simulink model "gm_commrshdl_ref"  (R2023b)
settings: Solver=FixedStepDiscrete  StartTime=0.0  StopTime=2100  RelTol=1e-3
InitFcn:
  | messagelength = 32;
  | period =messagelength+672;
  | N = 255;
  | K = 223;
  | 
  | message = [212 186 161 18 242 116 150 48 39 212 136 156 150 227 169 82 179 21 171 253 146 83 7 50 192 98 72 240 25 34 224 145 98 26 193 0];
libraries: simulink x9, whdlutilities x2, whdledac x1, hdlsllib x1
settings Model: ModifiedByFormat=The MathWorks Inc.  Creator=The MathWorks, Inc.  LastModifiedBy=The MathWorks Inc.
settings SolverCC: AlgebraicLoopSolver=TrustRegion
settings DataIOCC: LimitDataPoints=on  SaveFormat=Array  SaveOutput=off  SaveTime=off  ReturnWorkspaceOutputs=off  SignalLoggingName=RS_HDL_logsout
settings OptimizationCC: BlockReduction=off  ConditionallyExecuteInputs=off  DefaultParameterBehavior=Inlined  InheritOutputTypeSmallerThanSingle=on  OptimizeBlockIOStorage=off  ExpressionDepthLimit=2147483647
settings DebuggingCC: AlgebraicLoopMsg=error  UnderspecifiedInitializationDetection=Classic  MergeDetectMultiDrivingBlocksExec=none  SolverPrmCheckMsg=warning  InheritedTsInSrcMsg=none  MultiTaskDSMMsg=warning  MultiTaskCondExecSysMsg=none  SingleTaskRateTransMsg=error  UnconnectedInputMsg=warning  UnconnectedOutputMsg=warning  UnconnectedLineMsg=warning  AllowSymbolicDim=off  StateNameClashWarn=warning  SymbolicDimsDataTypeCodeGenerationDiagnostic=none  SFUnexpectedBacktrackingDiag=warning  SFNoUnconditionalDefaultTransitionDiag=warning  SFExecutionAtInitializationDiag=none  ArithmeticOperatorsInVariantConditions=warning
settings HardwareCC: ProdBitPerPointer=32  ProdBitPerSizeT=32  ProdBitPerPtrDiffT=32  ProdLargestAtomicFloat=None  ProdIntDivRoundTo=Undefined  ProdEndianess=Unspecified  ProdWordSize=32  ProdHWDeviceType=ASIC/FPGA->ASIC/FPGA  TargetBitPerPointer=64  TargetBitPerSizeT=64  TargetBitPerPtrDiffT=64  TargetLongLongMode=on  TargetIntDivRoundTo=Zero  TargetEndianess=LittleEndian  TargetWordSize=64  TargetHWDeviceType=Generic->Custom  ProdEqTarget=off
settings ModelReferenceCC: EnableRefExpFcnMdlSchedulingChecks=on  PropagateSignalLabelsOutOfModel=off
settings SFSimCC: SimUseLocalCustomCode=off  CustomCodeUndefinedFunction=UseInterfaceOnly
settings RTWCC: Description=SystemVerilog DPI Component Generator  SystemTargetFile=systemverilog_dpi_grt.tlc  TemplateMakefile=systemverilog_dpi_grt_default_tmf  RTWVerbose=off  RTWUseLocalCustomCode=off  BuildConfiguration=Faster Runs
settings CodeAppCC: MaxIdLength=256  StateflowObjectComments=on
settings DPIGRTTargetCC: TargetFcnLib=ansi_tfl_table_tmw.mat  GenFloatMathFcnCalls=NOT IN USE  TargetLangStandard=C99 (ISO)  CodeReplacementLibrary=None  UtilityFuncGeneration=Auto  MultiwordTypeDef=System defined  MultiwordLength=2048  DynamicStringBufferSize=256  GenerateFullHeader=on  InferredTypesCompatibility=off  GenerateSampleERTMain=off  GenerateTestInterfaces=off  ModelReferenceCompliant=on  ParMdlRefBuildCompliant=on  CompOptLevelCompliant=off  ConcurrentExecutionCompliant=off  IncludeMdlTerminateFcn=on  CombineOutputUpdateFcns=off  CombineSignalStateStructs=on  GroupInternalDataByFunction=off  SuppressErrorStatus=off  IncludeFileDelimiter=Auto  ERTCustomFileBanners=off  SupportAbsoluteTime=on  LogVarNameModifier=rt_  MatFileLogging=off  CodeInterfacePackaging=Reusable function  PurelyIntegerCode=off  SupportNonFinite=on  SupportComplex=on  SupportContinuousTime=on  SupportNonInlinedSFcns=on  RemoveDisableFunc=off  RemoveResetFunc=off  SupportVariableSizeSignals=off  ParenthesesLevel=Nominal  CastingMode=Nominal  MATLABClassNameForMDSCustomization=Simulink.SoftwareTarget.TargetSpecificTriggerConfigurationBase  ModelStepFunctionPrototypeControlCompliant=off  CPPClassGenCompliant=off  AutosarCompliant=off  MDXCompliant=off  GRTInterface=off  GenerateAllocFcn=on  UseToolchainInfoCompliant=on  GenerateSharedConstants=on  CoderGroups=[]  AccessMethods=[]  LookupTableObjectStructAxisOrder=1,2,3,4,...  LUTObjectStructOrderExplicitValues=Size,Breakpoints,Table  LUTObjectStructOrderEvenSpacing=Size,Breakpoints,Table  ArrayLayout=Column-major  UnsupportedSFcnMsg=error  ERTHeaderFileRootName=$R$E  ERTSourceFileRootName=$R$E  ERTDataFileRootName=$R_data  OptimizeReductions=off  RTWCAPISignals=on  RTWCAPIParams=off  RTWCAPIStates=off  RTWCAPIRootIO=off  ExtMode=off  ExtModeTransport=0  ExtModeStaticAlloc=off  ExtModeStaticAllocSize=1000000  ExtModeTesting=off  ExtModeMexFile=ext_comm  GenerateASAP2=off  MultiInstanceErrorCode=Error  DPICustomizeSystemVerilogCode=on  DPISystemVerilogTemplate=hdlverifier_dpitb_template.vgt  DPIReportRunTimeError=off  DPIRunTimeErrorSeverity=Fatal  DPIScalarizePorts=off  DPIGenerateTestBench=off  DPITestBenchSimulator=Mentor Graphics Questasim  DPITestPointAccessFcnInterface=None  DPIFixedPointDataType=CompatibleCType  DPIPortConnection=Port list  DPICompositeDataType=Flattened  DPIComponentTemplateType=Sequential
settings ConfigComp: CovMetricSettings=dw  CovSaveCumulativeToWorkspaceVar=on  CovSaveSingleToWorkspaceVar=on  CovExternalEMLEnable=off  CovSFcnEnable=off

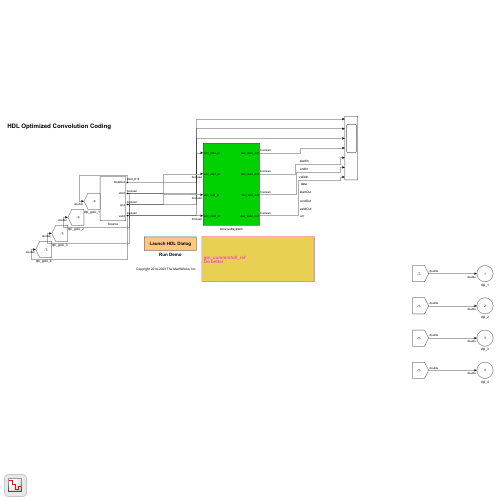
[thumbnail: Simulink's stored preview of the top-level diagram]
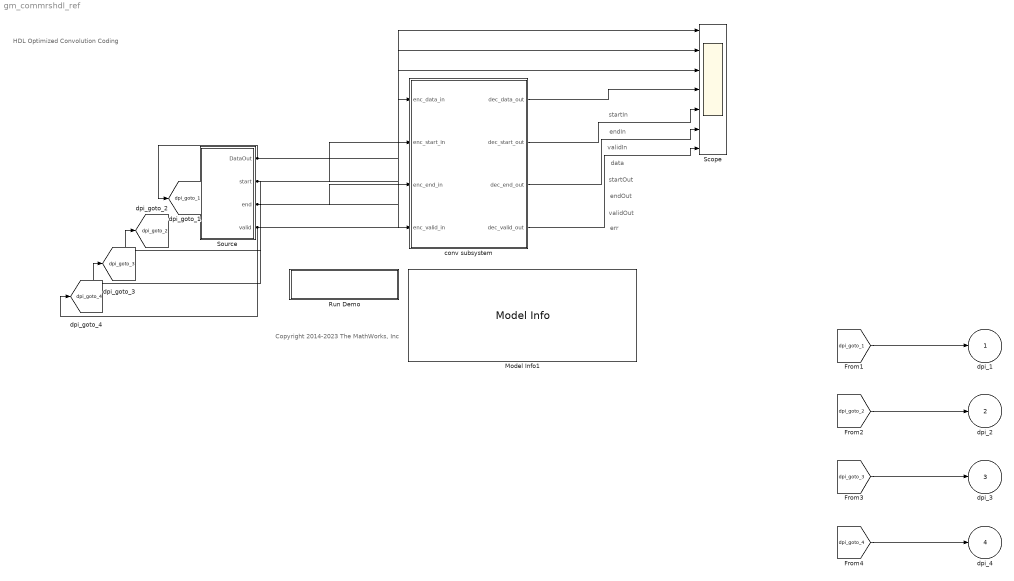
== system gm_commrshdl_ref ==
  note: err
  note: validOut
  note: endOut
  note: startOut
  note: data
  note: validIn
  note: endIn
  note: startIn
  note: Copyright 2014-2023 The MathWorks, Inc
  note: HDL Optimized Convolution Coding
  Model Info1 : simulink/Model-Wide Utilities/Model Info  Frame=on  DisplayStringWithTags=|  HorizontalTextAlignment=Left  LeftAlignmentValue=0.02
      | %<ModelName>
      | Do better
  Run Demo : Subsystem
      settings: OpenFcn=hdldialog(bdroot)
      mask Display: disp('Launch HDL Dialog')
  Scope : Scope  NumInputPorts=7
  Source : Subsystem
  conv subsystem : Subsystem
  dpi_1 : Outport
  dpi_2 : Outport  Port=2
  dpi_3 : Outport  Port=3
  dpi_4 : Outport  Port=4
  tag scope: dpi_goto_1=global, dpi_goto_2=global, dpi_goto_3=global, dpi_goto_4=global
  wires:
  Source/2(start) -> conv subsystem/2(enc_start_in), Scope/1, [dpi_goto_2]
  Source/3(end) -> conv subsystem/3(enc_end_in), Scope/2, [dpi_goto_3]
  Source/4(valid) -> conv subsystem/4(enc_valid_in), Scope/3, [dpi_goto_4]
  conv subsystem/1(dec_data_out) -> Scope/4
  conv subsystem/4(dec_valid_out) -> Scope/7
  conv subsystem/3(dec_end_out) -> Scope/6
  conv subsystem/2(dec_start_out) -> Scope/5
  Source/1(DataOut) -> conv subsystem/1(enc_data_in), [dpi_goto_1]
  [dpi_goto_1] -> dpi_1/1
  [dpi_goto_2] -> dpi_2/1
  [dpi_goto_3] -> dpi_3/1
  [dpi_goto_4] -> dpi_4/1

== system gm_commrshdl_ref/Run Demo ==

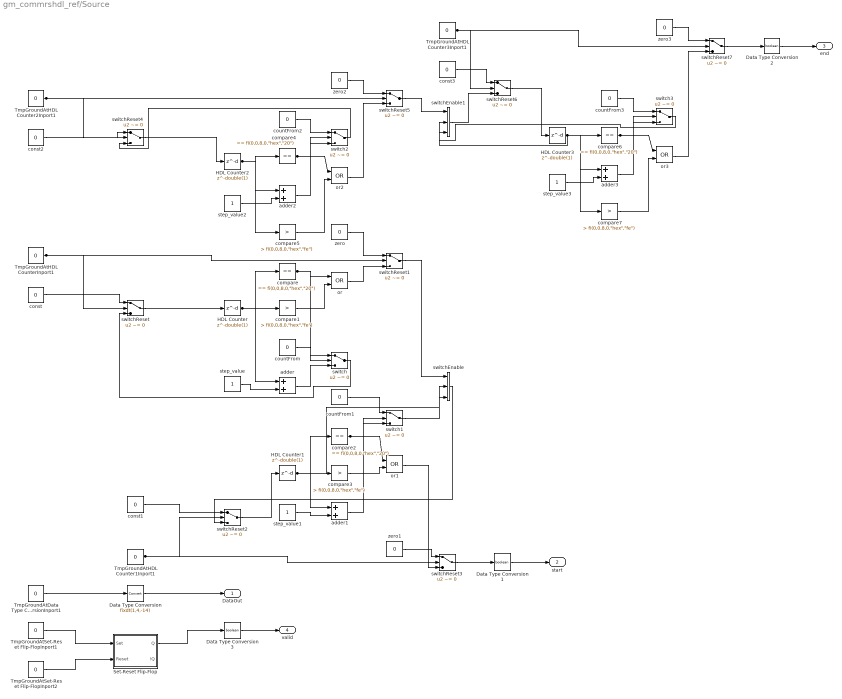
== system gm_commrshdl_ref/Source ==
  Data Type Conversion : DataTypeConversion  OutDataTypeStr=fixdt(1,4,-14)
  Data Type Conversion1 : DataTypeConversion  OutDataTypeStr=boolean
  Data Type Conversion2 : DataTypeConversion  OutDataTypeStr=boolean
  Data Type Conversion3 : DataTypeConversion  OutDataTypeStr=boolean
  HDL Counter{,1..3} (4 alike) : Delay  DelayLength=double(1)  InitialCondition=0  SampleTime=42
  Set-Reset Flip-Flop : Subsystem  mask(Set-Reset Flip-Flop){UndefState=Set, Q0=double(0), Ts=double(-1)}
      mask prompts: UndefState "physmod:ee:library:comments:control:eeGeneralControl:PriorityWhenUndefinedState_MP"; Q0 "physmod:ee:library:comments:control:eeGeneralControl:InitialConditionForQState_MP"; Ts "physmod:ee:library:comments:control:eeGeneralControl:SampleTime1ForInherited_MP"
      mask help: physmod:ee:library:comments:control:eeGeneralControl:SetResetFlipFlop_MD
      mask init:
      | Q0 = double(0);
      | Ts = double(-1);
      | UndefState = double(2);
      | isSetWhenUndefinedState = double(1);
      | timeDomain = 'Discrete';
      mask Help: web(nesl_help(gcbh))
      mask TypeOptions UndefState: physmod:ee:library:comments:control:eeGeneralControl:Reset_PV | physmod:ee:library:comments:control:eeGeneralControl:Set_PV
      mask Display: ee.mask.drawSetResetFlipFlop;
  TmpGroundAtData Type ConversionInport1 : Constant  Value=0  VectorParams1D=off  OutDataTypeStr=fixdt(1, 4, -14)
  TmpGroundAtHDL Counter1Inport1 : Constant  Value=0  VectorParams1D=off  OutDataTypeStr=boolean
  TmpGroundAtHDL Counter2Inport1 : Constant  Value=0  VectorParams1D=off  OutDataTypeStr=boolean
  TmpGroundAtHDL Counter3Inport1 : Constant  Value=0  VectorParams1D=off  OutDataTypeStr=boolean
  TmpGroundAtHDL CounterInport1 : Constant  Value=0  VectorParams1D=off  OutDataTypeStr=boolean
  TmpGroundAtSet-Reset Flip-FlopInport1 : Constant  Value=0  VectorParams1D=off  OutDataTypeStr=boolean
  TmpGroundAtSet-Reset Flip-FlopInport2 : Constant  Value=0  VectorParams1D=off  OutDataTypeStr=boolean
  adder{,1..3} (4 alike) : Sum  OutDataTypeStr=uint8  AccumDataTypeStr=uint8  SampleTime=42
  compare{,2,4,6} (4 alike) : simulink/Logic and Bit Operations/Compare To Constant  relop===  const="fi(0,0,8,0,\"hex\",\"20\")"  OutDataTypeStr=boolean
  compare{1,3,5,7} (4 alike) : simulink/Logic and Bit Operations/Compare To Constant  relop=>  const="fi(0,0,8,0,\"hex\",\"fe\")"  OutDataTypeStr=boolean
  const{,1..3} (4 alike) : Constant  Value=0  VectorParams1D=off  OutDataTypeStr=uint8  SampleTime=42
  countFrom{,1..3} (4 alike) : Constant  Value=0  VectorParams1D=off  OutDataTypeStr=uint8  SampleTime=42
  or{,1..3} (4 alike) : Logic  Operator=OR  AllPortsSameDT=off  OutDataTypeStr=boolean  SampleTime=42
  step_value{,1..3} (4 alike) : Constant  VectorParams1D=off  OutDataTypeStr=uint8  SampleTime=42
  switch{,1..3} (4 alike) : Switch  Criteria=u2 ~= 0  Threshold=double(0)  OutDataTypeStr=uint8  SampleTime=42  SaturateOnIntegerOverflow=off  InputSameDT=off
  switchEnable : MultiPortSwitch  DataPortOrder=Zero-based contiguous  Inputs=2  DiagnosticForDefault=None  zeroidx=on  OutDataTypeStr=uint8  SampleTime=42  SaturateOnIntegerOverflow=off  InputSameDT=off
  switchEnable1 : MultiPortSwitch  DataPortOrder=Zero-based contiguous  Inputs=2  DiagnosticForDefault=None  zeroidx=on  OutDataTypeStr=uint8  SampleTime=42  SaturateOnIntegerOverflow=off  InputSameDT=off
  switchReset{,2,4,6} (4 alike) : Switch  Criteria=u2 ~= 0  Threshold=double(0)  OutDataTypeStr=uint8  SampleTime=42  SaturateOnIntegerOverflow=off  InputSameDT=off
  switchReset{1,3,5,7} (4 alike) : Switch  Criteria=u2 ~= 0  Threshold=double(0)  OutDataTypeStr=boolean  SampleTime=42  SaturateOnIntegerOverflow=off  InputSameDT=off
  zero{,1..3} (4 alike) : Constant  Value=0  VectorParams1D=off  OutDataTypeStr=boolean  SampleTime=42
  DataOut : Outport  VectorParamsAs1DForOutWhenUnconnected=off
  start : Outport  Port=2  SampleTime=42  VectorParamsAs1DForOutWhenUnconnected=off
  end : Outport  Port=3  SampleTime=42  VectorParamsAs1DForOutWhenUnconnected=off
  valid : Outport  Port=4  SampleTime=42  VectorParamsAs1DForOutWhenUnconnected=off
  wires:
  zero3/1 -> switchReset7/1
  switchReset6/1 -> HDL Counter3/1
  switchEnable1/1 -> switchReset6/3
  compare7/1 -> or3/2
  compare6/1 -> switch3/2, or3/1
  switch3/1 -> switchEnable1/3
  countFrom3/1 -> switch3/1
  or3/1 -> switchReset7/3
  step_value3/1 -> adder3/2
  const3/1 -> switchReset6/1
  adder3/1 -> switch3/3
  switchReset7/1 -> Data Type Conversion2/1
  HDL Counter3/1 -> adder3/1, compare6/1, compare7/1, switchEnable1/2
  zero2/1 -> switchReset5/1
  switchReset4/1 -> HDL Counter2/1
  compare5/1 -> or2/2
  compare4/1 -> switch2/2, or2/1
  switch2/1 -> switchReset4/3
  countFrom2/1 -> switch2/1
  or2/1 -> switchReset5/3
  step_value2/1 -> adder2/2
  const2/1 -> switchReset4/1
  adder2/1 -> switch2/3
  switchReset5/1 -> switchEnable1/1
  HDL Counter2/1 -> adder2/1, compare4/1, compare5/1
  zero1/1 -> switchReset3/1
  switchReset2/1 -> HDL Counter1/1
  switchEnable/1 -> switchReset2/3
  compare3/1 -> or1/2
  compare2/1 -> switch1/2, or1/1
  switch1/1 -> switchEnable/3
  countFrom1/1 -> switch1/1
  or1/1 -> switchReset3/3
  step_value1/1 -> adder1/2
  const1/1 -> switchReset2/1
  adder1/1 -> switch1/3
  switchReset3/1 -> Data Type Conversion1/1
  HDL Counter1/1 -> adder1/1, compare2/1, compare3/1, switchEnable/2
  zero/1 -> switchReset1/1
  switchReset/1 -> HDL Counter/1
  compare1/1 -> or/2
  compare/1 -> switch/2, or/1
  switch/1 -> switchReset/3
  countFrom/1 -> switch/1
  or/1 -> switchReset1/3
  step_value/1 -> adder/2
  const/1 -> switchReset/1
  adder/1 -> switch/3
  switchReset1/1 -> switchEnable/1
  HDL Counter/1 -> adder/1, compare/1, compare1/1
  TmpGroundAtSet-Reset Flip-FlopInport2/1 -> Set-Reset Flip-Flop/2(Reset)
  TmpGroundAtSet-Reset Flip-FlopInport1/1 -> Set-Reset Flip-Flop/1(Set)
  TmpGroundAtHDL CounterInport1/1 -> switchReset/2, switchReset1/2
  TmpGroundAtHDL Counter3Inport1/1 -> switchReset6/2, switchReset7/2
  TmpGroundAtHDL Counter2Inport1/1 -> switchReset4/2, switchReset5/2
  TmpGroundAtHDL Counter1Inport1/1 -> switchReset2/2, switchReset3/2
  TmpGroundAtData Type ConversionInport1/1 -> Data Type Conversion/1
  Set-Reset Flip-Flop/1(Q) -> Data Type Conversion3/1
  Data Type Conversion3/1 -> valid/1
  Data Type Conversion2/1 -> end/1
  Data Type Conversion1/1 -> start/1
  Data Type Conversion/1 -> DataOut/1

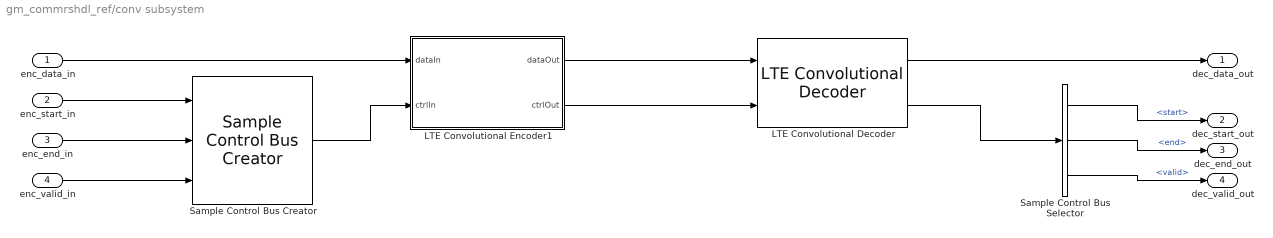
== system gm_commrshdl_ref/conv subsystem ==
  enc_data_in : Inport
  enc_start_in : Inport  Port=2  OutDataTypeStr=boolean
  enc_end_in : Inport  Port=3  OutDataTypeStr=boolean
  enc_valid_in : Inport  Port=4  OutDataTypeStr=boolean
  LTE Convolutional Decoder : whdledac/LTE Convolutional Decoder  MaximumMessageLength=1024  SimulateUsing=Code generation
  LTE Convolutional Encoder1 : Subsystem  AncestorBlock=whdledac/LTE Convolutional Encoder  mask(LTE Convolutional Encoder){BuffSize=1024}
      mask prompts: BuffSize "Maximum message length"
      mask help:
      | Implements a tailbiting convolutional encoder with the following parameters:
      | Rate 1/3
      | Constraint length 7
      | Octal code generator [133, 171, 165]
      mask init:
      | ltehdl.internal.ConvEncoderInit(gcb);
      mask DialogControl DescGroupVar Prompt: LTE Convolutional Encoder
      mask DialogControl DescTextVar Prompt: Implements a tailbiting convolutional encoder with the following parameters:
      mask DialogControl DescTextVar_copy Prompt: Rate 1/3
      mask DialogControl DescTextVar_copy_copy Prompt: Constraint length 7
      mask DialogControl DescTextVar_copy_copy_copy Prompt: Octal code generator [133, 171, 165]
      mask Display:
      | disp('LTE Convolutional\nEncoder');
      | port_label('input',1,'data');
      | port_label('input',2,'ctrl');
      | port_label('output',1,'data');
      | port_label('output',2,'ctrl');
  Sample Control Bus Creator : whdlutilities/Sample Control Bus Creator
  Sample Control Bus Selector : whdlutilities/Sample Control Bus Selector  OutputSignals=start,end,valid
  dec_data_out : Outport  VectorParamsAs1DForOutWhenUnconnected=off
  dec_start_out : Outport  Port=2  VectorParamsAs1DForOutWhenUnconnected=off
  dec_end_out : Outport  Port=3  VectorParamsAs1DForOutWhenUnconnected=off
  dec_valid_out : Outport  Port=4  VectorParamsAs1DForOutWhenUnconnected=off
  wires:
  enc_start_in/1 -> Sample Control Bus Creator/1
  enc_end_in/1 -> Sample Control Bus Creator/2
  enc_valid_in/1 -> Sample Control Bus Creator/3
  enc_data_in/1 -> LTE Convolutional Encoder1/1(dataIn)
  Sample Control Bus Creator/1 -> LTE Convolutional Encoder1/2(ctrlIn)
  LTE Convolutional Decoder/2 -> Sample Control Bus Selector/1
  LTE Convolutional Decoder/1 -> dec_data_out/1
  Sample Control Bus Selector/1 -> dec_start_out/1  "<start>"
  Sample Control Bus Selector/2 -> dec_end_out/1  "<end>"
  Sample Control Bus Selector/3 -> dec_valid_out/1  "<valid>"
  LTE Convolutional Encoder1/1(dataOut) -> LTE Convolutional Decoder/1
  LTE Convolutional Encoder1/2(ctrlOut) -> LTE Convolutional Decoder/2

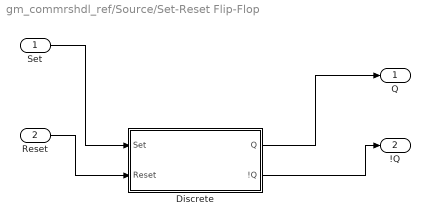
== system gm_commrshdl_ref/Source/Set-Reset Flip-Flop ==
  Set : Inport  OutDataTypeStr=boolean
  Reset : Inport  Port=2  OutDataTypeStr=boolean
  Discrete : Subsystem
  Q : Outport  SampleTime=42
  !Q : Outport  Port=2  SampleTime=42
  wires:
  Discrete/2(!Q) -> !Q/1
  Discrete/1(Q) -> Q/1
  Reset/1 -> Discrete/2(Reset)
  Set/1 -> Discrete/1(Set)

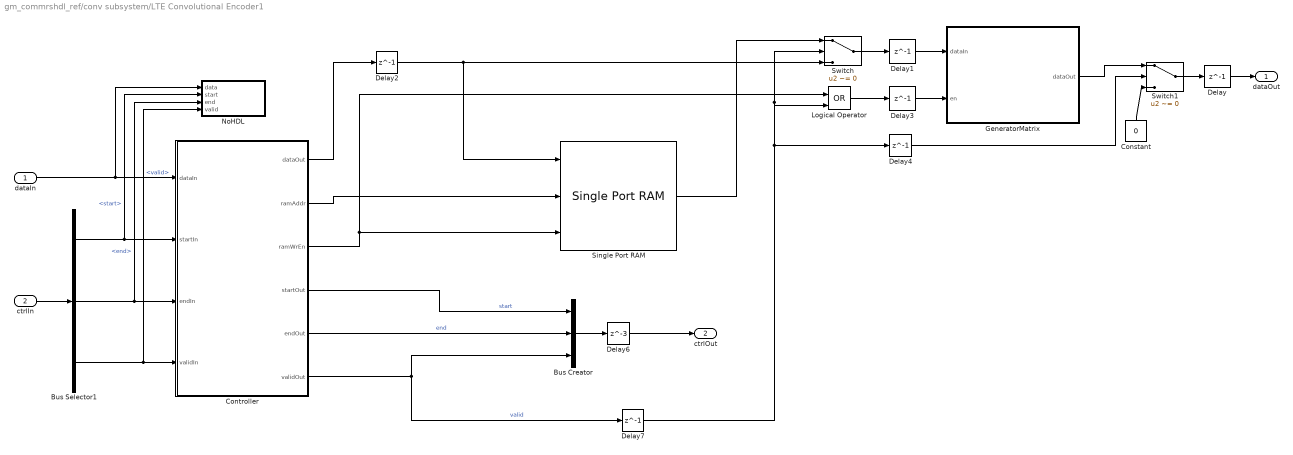
== system gm_commrshdl_ref/conv subsystem/LTE Convolutional Encoder1 ==
  dataIn : Inport
  ctrlIn : Inport  Port=2
  Bus Creator : BusCreator  Inputs=3  OutDataTypeStr=Bus: samplecontrol  NonVirtualBus=on
      mask init:
      | registersamplecontrolbus;
      settings: InheritFromInputs=off
  Bus Selector1 : BusSelector  OutputSignals=start,end,valid
  Constant : Constant  Value=0  OutDataTypeStr=boolean  SampleTime=-1
  Controller : MATLAB Function  TreatAsAtomicUnit=on
  Delay : Delay  DelayLength=1
  Delay1 : Delay  DelayLength=1
  Delay2 : Delay  DelayLength=1  InitialCondition=0  UseCircularBuffer=on
  Delay3 : Delay  DelayLength=1
  Delay4 : Delay  DelayLength=1  InitialCondition=0  UseCircularBuffer=on
  Delay6 : Delay  DelayLength=3  InitialCondition=0  UseCircularBuffer=on
  Delay7 : Delay  DelayLength=1  InitialCondition=0  UseCircularBuffer=on
  GeneratorMatrix : MATLAB Function  TreatAsAtomicUnit=on
  Logical Operator : Logic  Operator=OR  IconShape=distinctive  AllPortsSameDT=off  OutDataTypeStr=boolean
  NoHDL : Subsystem
  Single Port RAM : hdlsllib/HDL RAMs/Single Port RAM  ram_size=nextpow2(BuffSize)  dout_type=Old data
  Switch : Switch  Criteria=u2 ~= 0  SaturateOnIntegerOverflow=off  InputSameDT=off
  Switch1 : Switch  Criteria=u2 ~= 0  SaturateOnIntegerOverflow=off  InputSameDT=off
  dataOut : Outport  VectorParamsAs1DForOutWhenUnconnected=off
  ctrlOut : Outport  Port=2  VectorParamsAs1DForOutWhenUnconnected=off
  wires:
  Single Port RAM/1 -> Switch/1
  Delay7/1 -> Logical Operator/2, Switch/2, Delay4/1
  Delay6/1 -> ctrlOut/1
  Switch/1 -> Delay1/1
  Controller/6(validOut) -> Bus Creator/3, Delay7/1  "valid"
  Delay3/1 -> GeneratorMatrix/2(en)
  Constant/1 -> Switch1/3
  Controller/1(dataOut) -> Delay2/1
  GeneratorMatrix/1(dataOut) -> Switch1/1
  Delay4/1 -> Switch1/2
  Delay1/1 -> GeneratorMatrix/1(dataIn)
  Bus Selector1/1 -> NoHDL/2(start), Controller/2(startIn)  "<start>"
  Logical Operator/1 -> Delay3/1
  Controller/3(ramWrEn) -> Logical Operator/1, Single Port RAM/3
  ctrlIn/1 -> Bus Selector1/1
  Delay2/1 -> Switch/3, Single Port RAM/1
  Bus Selector1/3 -> NoHDL/4(valid), Controller/4(validIn)  "<valid>"
  Controller/5(endOut) -> Bus Creator/2  "end"
  Controller/4(startOut) -> Bus Creator/1  "start"
  Delay/1 -> dataOut/1
  Bus Selector1/2 -> NoHDL/3(end), Controller/3(endIn)  "<end>"
  Controller/2(ramAddr) -> Single Port RAM/2
  Bus Creator/1 -> Delay6/1
  dataIn/1 -> NoHDL/1(data), Controller/1(dataIn)
  Switch1/1 -> Delay/1

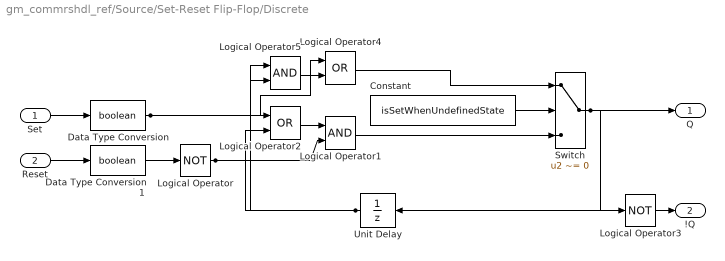
== system gm_commrshdl_ref/Source/Set-Reset Flip-Flop/Discrete ==
  Set : Inport  OutDataTypeStr=boolean  PortDimensions=1
  Reset : Inport  Port=2  OutDataTypeStr=boolean  PortDimensions=1
  Constant : Constant  Value=isSetWhenUndefinedState  SampleTime=Ts
  Data Type Conversion : DataTypeConversion  OutDataTypeStr=boolean  SaturateOnIntegerOverflow=off  RndMeth=Floor
  Data Type Conversion1 : DataTypeConversion  OutDataTypeStr=boolean  SaturateOnIntegerOverflow=off  RndMeth=Floor
  Logical Operator : Logic  Operator=NOT  AllPortsSameDT=off  OutDataTypeStr=boolean
  Logical Operator1 : Logic  AllPortsSameDT=off  OutDataTypeStr=boolean
  Logical Operator2 : Logic  Operator=OR  AllPortsSameDT=off  OutDataTypeStr=boolean
  Logical Operator3 : Logic  Operator=NOT  AllPortsSameDT=off  OutDataTypeStr=boolean
  Logical Operator4 : Logic  Operator=OR  AllPortsSameDT=off  OutDataTypeStr=boolean
  Logical Operator5 : Logic  AllPortsSameDT=off  OutDataTypeStr=boolean
  Switch : Switch  Criteria=u2 ~= 0  Threshold=1  SaturateOnIntegerOverflow=off  InputSameDT=off
  Unit Delay : UnitDelay  InitialCondition=Q0  SampleTime=-1  HasFrameUpgradeWarning=on
  Q : Outport  SampleTime=42  VectorParamsAs1DForOutWhenUnconnected=off
  !Q : Outport  Port=2  SampleTime=42  VectorParamsAs1DForOutWhenUnconnected=off
  wires:
  Unit Delay/1 -> Logical Operator2/2, Logical Operator5/2
  Switch/1 -> Q/1, Unit Delay/1, Logical Operator3/1
  Logical Operator5/1 -> Logical Operator4/2
  Logical Operator4/1 -> Switch/1
  Logical Operator3/1 -> !Q/1
  Logical Operator2/1 -> Logical Operator1/1
  Logical Operator1/1 -> Switch/3
  Logical Operator/1 -> Logical Operator1/2, Logical Operator5/1
  Data Type Conversion1/1 -> Logical Operator/1
  Data Type Conversion/1 -> Logical Operator2/1, Logical Operator4/1
  Constant/1 -> Switch/2
  Reset/1 -> Data Type Conversion1/1
  Set/1 -> Data Type Conversion/1

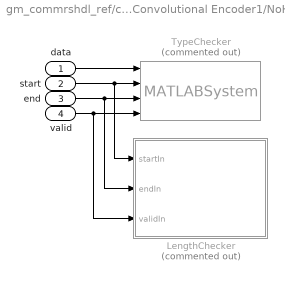
== system gm_commrshdl_ref/conv subsystem/LTE Convolutional Encoder1/NoHDL ==
  data : Inport
  start : Inport  Port=2
  end : Inport  Port=3
  valid : Inport  Port=4
  LengthChecker : MATLAB Function  Commented=on  TreatAsAtomicUnit=on
  TypeChecker : MATLABSystem  Commented=on  System=ltehdl.internal.ConvEncCheckType  SimulateUsing=Code generation
      mask Type: ltehdl.internal.ConvEncCheckType
      mask Display: disp('ConvEncCheckType');
  wires:
  end/1 -> LengthChecker/2(endIn), TypeChecker/3
  data/1 -> TypeChecker/1
  start/1 -> LengthChecker/1(startIn), TypeChecker/2
  valid/1 -> LengthChecker/3(validIn), TypeChecker/4

== matlab function gm_commrshdl_ref/conv subsystem/LTE Convolutional Encoder1/Controller ==
  settings: fimath=fimath('RoundingMethod', 'Floor','OverflowAction', 'Wrap','ProductMode', 'FullPrecision', 'SumMode', 'FullPrecision')
  data: dataIn input; dataOut output; startIn input; ramAddr output; endIn input; validIn input; ramWrEn output; startOut output; endOut output; validOut output; BuffSize parameter double
function [dataOut, ramAddr, ramWrEn, startOut, endOut, validOut] = Controller(dataIn,startIn,endIn,validIn, BuffSize)
    %#codegen
    
    % states
    ENC_IDLE          = 0;        % waiting for start
    ENC_STREAM_IN     = 1;        % streaming input and writing into RAM
    ENC_STREAM_IN_END = 2;        % last input bit
    ENC_STREAM_OUT    = 3;        % stream data out of RAM through encoder
    
    persistent encoderStateReg;   % current state of decoder
    persistent ramAddrReg;        % buffer write address
    persistent ramAddrEndReg;     % value at which rd_addr counter should stop counting
    persistent ramWrEnReg;        % buffer write enable
    persistent dataReg;
    
    if isempty(ramWrEnReg)
        encoderStateReg = fi(ENC_IDLE,0,2,0);
        ramAddrReg      = fi(0,0,nextpow2(BuffSize),0,'OverflowAction','Wrap');
        ramAddrEndReg   = fi(0,0,nextpow2(BuffSize),0,'OverflowAction','Wrap');
        ramWrEnReg      = false;
        if isa(dataIn,'embedded.fi')
            dataReg = fi(false(length(dataIn),1),dataIn.numerictype); %ufi(0,1,0);
        else
            dataReg = cast(zeros(length(dataIn),1),class(dataIn));
        end
    end
    
    % assign outputs
    if nextpow2(BuffSize) == 8
        ramAddr       = uint8(ramAddrReg);
    elseif nextpow2(BuffSize) == 16
        ramAddr       = uint16(ramAddrReg);
    else
        ramAddr       = ramAddrReg;
    end
    ramWrEn       = ramWrEnReg;
    startOut      = (encoderStateReg == ENC_STREAM_OUT) && (ramAddrReg == 0);
    endOut        = (encoderStateReg == ENC_STREAM_OUT) && (ramAddrReg == ramAddrEndReg);
    validOut      = (encoderStateReg == ENC_STREAM_OUT);
    %     ready         = (encoderStateReg == ENC_IDLE);
    
    %----------------------------------------------------------------------------------------------
    % synchronous logic
    %----------------------------------------------------------------------------------------------
    
    ramWrEnReg(:) = validIn && (startIn || (encoderStateReg == ENC_STREAM_IN));
    
    if (encoderStateReg == ENC_STREAM_IN_END)
        ramAddrEndReg(:) = ramAddrReg;
    end
    
    switch encoderStateReg
        case ENC_IDLE
            
            if validIn && startIn
                encoderStateReg(:) = ENC_STREAM_IN;
                ramAddrReg(:)      = 0;
            end
            
        case ENC_STREAM_IN
            
            if validIn
                if endIn
                    encoderStateReg(:) = ENC_STREAM_IN_END;
                    ramAddrReg(:)      = ramAddrReg + 1;
                elseif startIn
                    encoderStateReg(:) = ENC_STREAM_IN;
                    ramAddrReg(:) = 0;
                else
                    encoderStateReg(:) = ENC_STREAM_IN;
                    ramAddrReg(:)      = ramAddrReg + 1;
                end
            end
            
        case ENC_STREAM_IN_END
            
            %             encoderStateReg(:) = ENC_STREAM_OUT;
            ramAddrReg(:)      = 0;
            if validIn && startIn
                encoderStateReg(:) = ENC_STREAM_IN;
            else
                encoderStateReg(:) = ENC_STREAM_OUT;
            end
            
        case ENC_STREAM_OUT
            
            if validIn && startIn
                ramAddrReg(:) = 0;
                encoderStateReg(:) = ENC_STREAM_IN;
            else
                if (ramAddrReg == ramAddrEndReg)
                    encoderStateReg(:) = ENC_IDLE;
                    ramAddrReg(:)      = 0;
                else
                    encoderStateReg(:) = ENC_STREAM_OUT;
                    ramAddrReg(:)      = ramAddrReg + 1;
                end
            end
    end
    
    dataReg(:) = dataIn;
    dataOut = dataIn(1);
    
end

== matlab function gm_commrshdl_ref/conv subsystem/LTE Convolutional Encoder1/GeneratorMatrix ==
  settings: fimath=fimath('RoundingMethod', 'Floor','OverflowAction', 'Wrap','ProductMode', 'FullPrecision', 'SumMode', 'FullPrecision')
  data: dataIn input; dataOut output; en input
function dataOut  = FunctionGenerator(dataIn,en)
    %#codegen
    
    G_value = [...
        1 0 1 1 0 1 1;
        1 1 1 1 0 0 1;
        1 1 1 0 1 0 1];
    
    localFimath = fimath(...
        'OverflowAction', 'Wrap', ...
        'ProductMode', 'SpecifyPrecision', ...
        'ProductWordLength', 1, ...
        'ProductFractionLength', 0, ...
        'SumMode', 'SpecifyPrecision', ...
        'SumWordLength', 1, ...
        'SumFractionLength', 0);
    
    G = fi(G_value, 0, 1, 0, localFimath);
    
    % current state of decoder
    persistent shiftReg;
    
    if isempty(shiftReg)
        shiftReg = fi(zeros(7,1), 0, 1, 0, localFimath);
    end
    
    % shift register
    shiftRegNext = shiftReg;
    if en
        shiftRegNext = [cast(dataIn,'like',shiftReg); shiftReg(1:6)];
    end
    
    % compute function output
    dataOut = G * shiftRegNext;
    
    shiftReg = shiftRegNext;
    
end

== matlab function gm_commrshdl_ref/conv subsystem/LTE Convolutional Encoder1/NoHDL/LengthChecker ==
  settings: fimath=fimath('RoundingMethod', 'Floor','OverflowAction', 'Wrap','ProductMode', 'FullPrecision', 'SumMode', 'FullPrecision')
  data: startIn input; endIn input; validIn input; BuffSize parameter
function checkMsgLength(startIn,endIn,validIn, BuffSize)
    % Check the length of frame if matches the LTE standard.
    
    WAIT_S = ufi(0,2,0);
    COUNT_S = ufi(1,2,0);
    RST_S = ufi(2,2,0);
    
    persistent lenState;
    persistent lenCounter;
    
    if isempty(lenState)
        lenState= WAIT_S;
        lenCounter = ufi(0,17,0);
    end
    
    nextLenState   = lenState;
    nextLenCounter = lenCounter;
    
    switch(lenState)
        case WAIT_S
            nextLenCounter(:) = 0;
            if startIn && validIn
                nextLenState = COUNT_S;
            else
                nextLenState = WAIT_S;
            end
            
        case COUNT_S
            if validIn
                if endIn
                    nextLenCounter(:) = lenCounter + 1;
                    nextLenState = RST_S;
                elseif startIn
                    nextLenCounter(:) = 0;
                else
                    nextLenCounter(:) = lenCounter + 1;
                end
            end
        otherwise
            if validIn && startIn
                nextLenState = COUNT_S;
                nextLenCounter(:) = 0;
            else
                nextLenState = WAIT_S;
            end
    end
    
    if (nextLenCounter <5 || nextLenCounter > BuffSize-1) && (endIn == true) && nextLenState == RST_S
        coder.internal.warning('whdl:ConvolutionalCode:InvalidDataLength',int2str(double(nextLenCounter+1)));
    end
    
    lenState   = nextLenState;
    lenCounter = nextLenCounter;
    
end
